simulink model "C_LQR"  (R2020b)
settings: Solver=VariableStepAuto  StartTime=0.0  StopTime=30  RelTol=1e-3
values from neighbouring files (symbols this model uses):
  sysE = ss(tf(48*(Kt/Ra)))    [C_Hinf.m]
  sysM = ss(tf(Ra,[Ra*J Ke*Kt+Ra*B 0]))    [C_Hinf.m]
undefined symbols (not defined in the file or in its folder): K1, K2, K3, K4, K5
settings Model: Creator=andre  LastModifiedBy=andre

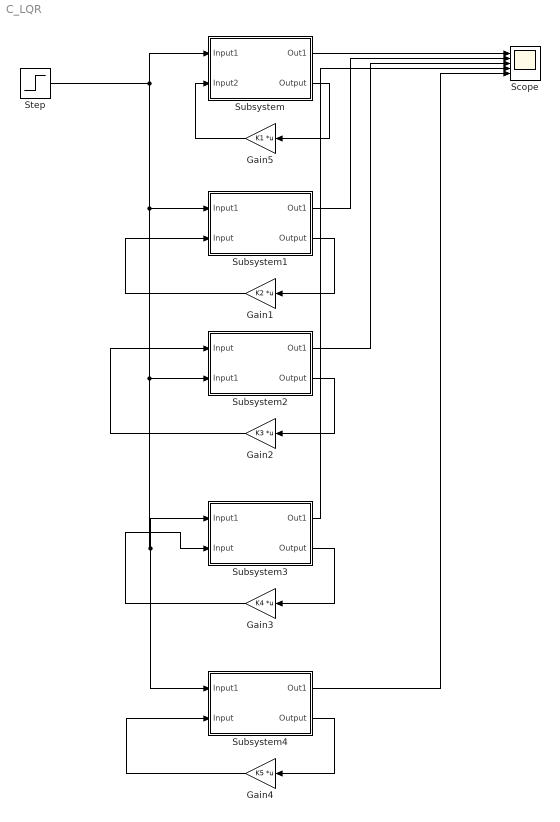
== system C_LQR ==
  Gain1 : Gain  Gain=K2  Multiplication=Matrix(K*u) (u vector)
  Gain2 : Gain  Gain=K3  Multiplication=Matrix(K*u) (u vector)
  Gain3 : Gain  Gain=K4  Multiplication=Matrix(K*u) (u vector)
  Gain4 : Gain  Gain=K5  Multiplication=Matrix(K*u) (u vector)
  Gain5 : Gain  Gain=K1  Multiplication=Matrix(K*u) (u vector)
  Scope : Scope  NumInputPorts=5
  Step : Step  Time=10  After=0.5  SampleTime=0
  Subsystem : Subsystem
  Subsystem1 : Subsystem
  Subsystem2 : Subsystem
  Subsystem3 : Subsystem
  Subsystem4 : Subsystem
  wires:
  Gain5/1 -> Subsystem/2(Input2)
  Subsystem/1(Out1) -> Scope/1
  Subsystem/2(Output) -> Gain5/1
  Gain1/1 -> Subsystem1/2(Input)
  Subsystem1/2(Output) -> Gain1/1
  Subsystem1/1(Out1) -> Scope/2
  Gain2/1 -> Subsystem2/1(Input)
  Subsystem2/2(Output) -> Gain2/1
  Subsystem2/1(Out1) -> Scope/3
  Gain3/1 -> Subsystem3/2(Input)
  Subsystem3/2(Output) -> Gain3/1
  Subsystem3/1(Out1) -> Scope/4
  Step/1 -> Subsystem4/1(Input1), Subsystem3/1(Input1), Subsystem2/2(Input1), Subsystem1/1(Input1), Subsystem/1(Input1)
  Gain4/1 -> Subsystem4/2(Input)
  Subsystem4/2(Output) -> Gain4/1
  Subsystem4/1(Out1) -> Scope/5

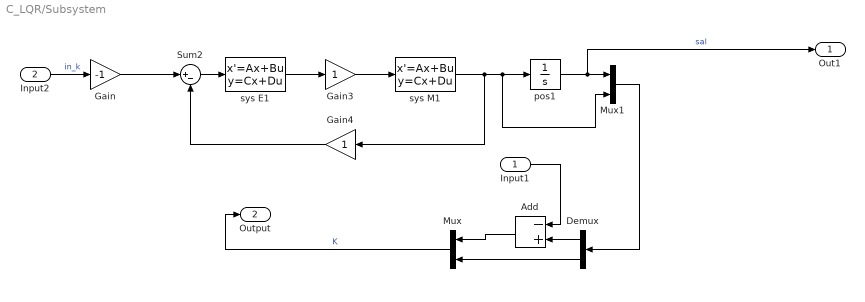
== system C_LQR/Subsystem ==
  Input1 : Inport
  Input2 : Inport  Port=2
  Add : Sum  Inputs=-+
  Demux : Demux  Outputs=2
  Gain : Gain  Gain=-1
  Gain3 : Gain
  Gain4 : Gain
  Mux : Mux  Inputs=2
  Mux1 : Mux  Inputs=2
  Sum2 : Sum  Inputs=|+-
  pos1 : Integrator  InitialCondition=1
  sys E1 : StateSpace  A=sysE.A  B=sysE.B  C=sysE.C  D=sysE.D  InitialCondition=0
  sys M1 : StateSpace  A=sysM.A  B=sysM.B  C=sysM.C  D=sysM.D  InitialCondition=0
  Out1 : Outport
  Output : Outport  Port=2
  wires:
  sys E1/1 -> Gain3/1
  sys M1/1 -> Mux1/2, pos1/1, Gain4/1
  Gain4/1 -> Sum2/2
  Mux/1 -> Output/1  "K"
  Demux/1 -> Add/2
  Gain3/1 -> sys M1/1
  Sum2/1 -> sys E1/1
  Add/1 -> Mux/1
  pos1/1 -> Out1/1, Mux1/1  "sal"
  Mux1/1 -> Demux/1
  Input1/1 -> Add/1
  Demux/2 -> Mux/2
  Gain/1 -> Sum2/1
  Input2/1 -> Gain/1  "in_k"

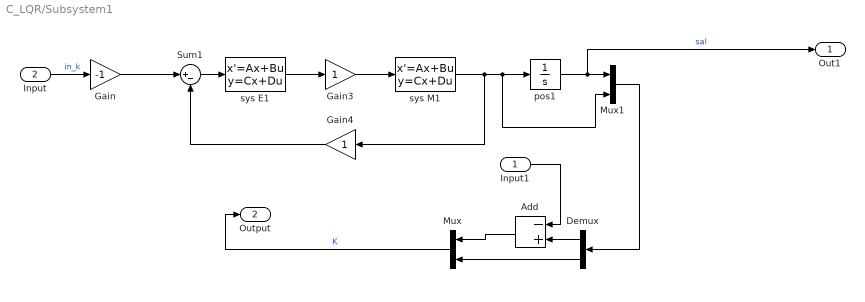
== system C_LQR/Subsystem1 ==
  Input1 : Inport
  Input : Inport  Port=2
  Add : Sum  Inputs=-+
  Demux : Demux  Outputs=2
  Gain : Gain  Gain=-1
  Gain3 : Gain
  Gain4 : Gain
  Mux : Mux  Inputs=2
  Mux1 : Mux  Inputs=2
  Sum1 : Sum  Inputs=|+-
  pos1 : Integrator  InitialCondition=1
  sys E1 : StateSpace  A=sysE.A  B=sysE.B  C=sysE.C  D=sysE.D  InitialCondition=0
  sys M1 : StateSpace  A=sysM.A  B=sysM.B  C=sysM.C  D=sysM.D  InitialCondition=0
  Out1 : Outport
  Output : Outport  Port=2
  wires:
  sys E1/1 -> Gain3/1
  sys M1/1 -> Mux1/2, pos1/1, Gain4/1
  Gain4/1 -> Sum1/2
  Mux/1 -> Output/1  "K"
  Demux/1 -> Add/2
  Gain3/1 -> sys M1/1
  Sum1/1 -> sys E1/1
  Add/1 -> Mux/1
  pos1/1 -> Out1/1, Mux1/1  "sal"
  Mux1/1 -> Demux/1
  Input1/1 -> Add/1
  Demux/2 -> Mux/2
  Gain/1 -> Sum1/1
  Input/1 -> Gain/1  "in_k"

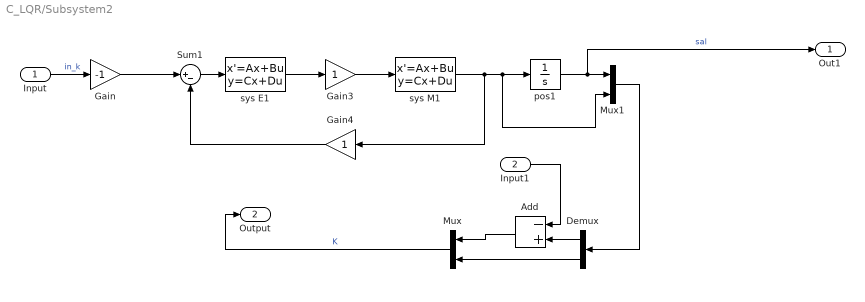
== system C_LQR/Subsystem2 ==
  Input : Inport
  Input1 : Inport  Port=2
  Add : Sum  Inputs=-+
  Demux : Demux  Outputs=2
  Gain : Gain  Gain=-1
  Gain3 : Gain
  Gain4 : Gain
  Mux : Mux  Inputs=2
  Mux1 : Mux  Inputs=2
  Sum1 : Sum  Inputs=|+-
  pos1 : Integrator  InitialCondition=1
  sys E1 : StateSpace  A=sysE.A  B=sysE.B  C=sysE.C  D=sysE.D  InitialCondition=0
  sys M1 : StateSpace  A=sysM.A  B=sysM.B  C=sysM.C  D=sysM.D  InitialCondition=0
  Out1 : Outport
  Output : Outport  Port=2
  wires:
  sys E1/1 -> Gain3/1
  sys M1/1 -> Mux1/2, pos1/1, Gain4/1
  Gain4/1 -> Sum1/2
  Mux/1 -> Output/1  "K"
  Demux/1 -> Add/2
  Input/1 -> Gain/1  "in_k"
  Gain3/1 -> sys M1/1
  Sum1/1 -> sys E1/1
  Add/1 -> Mux/1
  pos1/1 -> Out1/1, Mux1/1  "sal"
  Mux1/1 -> Demux/1
  Input1/1 -> Add/1
  Demux/2 -> Mux/2
  Gain/1 -> Sum1/1

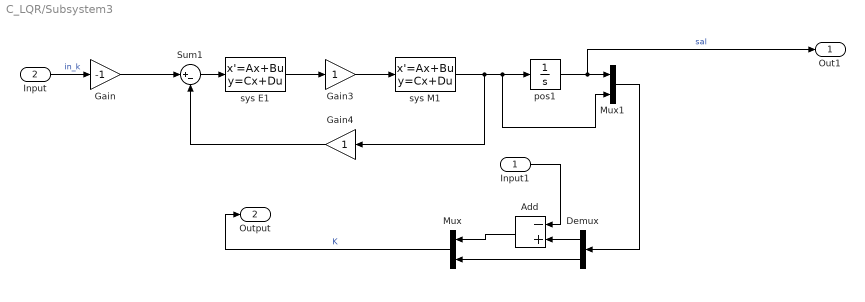
== system C_LQR/Subsystem3 ==
  Input1 : Inport
  Input : Inport  Port=2
  Add : Sum  Inputs=-+
  Demux : Demux  Outputs=2
  Gain : Gain  Gain=-1
  Gain3 : Gain
  Gain4 : Gain
  Mux : Mux  Inputs=2
  Mux1 : Mux  Inputs=2
  Sum1 : Sum  Inputs=|+-
  pos1 : Integrator  InitialCondition=1
  sys E1 : StateSpace  A=sysE.A  B=sysE.B  C=sysE.C  D=sysE.D  InitialCondition=0
  sys M1 : StateSpace  A=sysM.A  B=sysM.B  C=sysM.C  D=sysM.D  InitialCondition=0
  Out1 : Outport
  Output : Outport  Port=2
  wires:
  sys E1/1 -> Gain3/1
  sys M1/1 -> Mux1/2, pos1/1, Gain4/1
  Gain4/1 -> Sum1/2
  Mux/1 -> Output/1  "K"
  Demux/1 -> Add/2
  Gain3/1 -> sys M1/1
  Sum1/1 -> sys E1/1
  Add/1 -> Mux/1
  pos1/1 -> Out1/1, Mux1/1  "sal"
  Mux1/1 -> Demux/1
  Input1/1 -> Add/1
  Demux/2 -> Mux/2
  Gain/1 -> Sum1/1
  Input/1 -> Gain/1  "in_k"

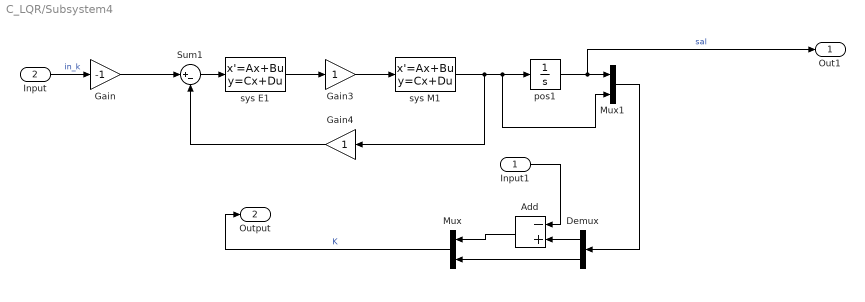
== system C_LQR/Subsystem4 ==
  Input1 : Inport
  Input : Inport  Port=2
  Add : Sum  Inputs=-+
  Demux : Demux  Outputs=2
  Gain : Gain  Gain=-1
  Gain3 : Gain
  Gain4 : Gain
  Mux : Mux  Inputs=2
  Mux1 : Mux  Inputs=2
  Sum1 : Sum  Inputs=|+-
  pos1 : Integrator  InitialCondition=1
  sys E1 : StateSpace  A=sysE.A  B=sysE.B  C=sysE.C  D=sysE.D  InitialCondition=0
  sys M1 : StateSpace  A=sysM.A  B=sysM.B  C=sysM.C  D=sysM.D  InitialCondition=0
  Out1 : Outport
  Output : Outport  Port=2
  wires:
  sys E1/1 -> Gain3/1
  sys M1/1 -> Mux1/2, pos1/1, Gain4/1
  Gain4/1 -> Sum1/2
  Mux/1 -> Output/1  "K"
  Demux/1 -> Add/2
  Gain3/1 -> sys M1/1
  Sum1/1 -> sys E1/1
  Add/1 -> Mux/1
  pos1/1 -> Out1/1, Mux1/1  "sal"
  Mux1/1 -> Demux/1
  Input1/1 -> Add/1
  Demux/2 -> Mux/2
  Gain/1 -> Sum1/1
  Input/1 -> Gain/1  "in_k"
